simulink model "dcmotor_model"  (R2018b)
settings: Solver=ode15s  StartTime=0.0  StopTime=10.0  RelTol=1e-3  EnableMultiTasking=on
values from neighbouring files (symbols this model uses):
  fm = 7.2702e-06    [init.m]
  Imax = 10    [init.m]
  Jm = 2.7438e-06    [init.m]
  k = 43.8    [init.m]
  kM = 0.0054436    [init.m]
  L = 2.2223e-05    [init.m]
  R = 4.0191    [init.m]
settings Model: Creator=Akos  LastModifiedBy=akos
settings OptimizationCC: LifeSpan=inf
settings DebuggingCC: SFUnexpectedBacktrackingDiag=warning  SFNoUnconditionalDefaultTransitionDiag=warning
settings SFSimCC: SimUseLocalCustomCode=off
settings RTWCC: RTWUseLocalCustomCode=off
settings CodeAppCC: StateflowObjectComments=on
settings GRTTargetCC: TargetLangStandard=C89/C90 (ANSI)
settings ConfigComp: CovMetricSettings=dw  CovHtmlReporting=on  CovSaveCumulativeToWorkspaceVar=on  CovSaveSingleToWorkspaceVar=on  CovExternalEMLEnable=off

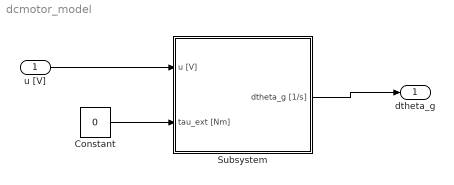
== system dcmotor_model ==
  u [V] : Inport
  Constant : Constant  Value=0
  Subsystem : Subsystem
  dtheta_g : Outport
  wires:
  u [V]/1 -> Subsystem/1(u [V])
  Constant/1 -> Subsystem/2(tau_ext [Nm])
  Subsystem/1(dtheta_g [1/s]) -> dtheta_g/1

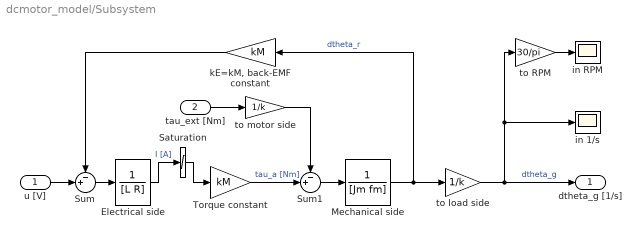
== system dcmotor_model/Subsystem ==
  u [V] : Inport
  tau_ext [Nm] : Inport  Port=2
  Electrical side : TransferFcn  Denominator=[L R]
  Mechanical side : TransferFcn  Denominator=[Jm fm]
  Saturation : Saturate  UpperLimit=Imax  LowerLimit=-Imax
  Sum : Sum  Inputs=-+|
  Sum1 : Sum  Inputs=-+|
  Torque constant : Gain  Gain=kM  SaturateOnIntegerOverflow=on  OutDataTypeStr=Inherit: Same as input  ParamDataTypeStr=Inherit: Same as input
  in 1/s : Scope
  in RPM : Scope
  "kE=kM, back-EMF constant" : Gain  Gain=kM  SaturateOnIntegerOverflow=on  OutDataTypeStr=Inherit: Same as input  ParamDataTypeStr=Inherit: Same as input
  to RPM : Gain  Gain=30/pi  SaturateOnIntegerOverflow=on  OutDataTypeStr=Inherit: Same as input  ParamDataTypeStr=Inherit: Same as input
  to load side : Gain  Gain=1/k  SaturateOnIntegerOverflow=on  OutDataTypeStr=Inherit: Same as input  ParamDataTypeStr=Inherit: Same as input
  to motor side : Gain  Gain=1/k  SaturateOnIntegerOverflow=on  OutDataTypeStr=Inherit: Same as input  ParamDataTypeStr=Inherit: Same as input
  dtheta_g [1/s] : Outport
  wires:
  tau_ext [Nm]/1 -> to motor side/1
  Sum/1 -> Electrical side/1
  to motor side/1 -> Sum1/1
  Torque constant/1 -> Sum1/2  "tau_a [Nm]"
  to load side/1 -> to RPM/1, in 1/s/1, dtheta_g [1/s]/1  "dtheta_g"
  "kE=kM, back-EMF constant"/1 -> Sum/1
  u [V]/1 -> Sum/2
  Sum1/1 -> Mechanical side/1
  Mechanical side/1 -> to load side/1, "kE=kM, back-EMF constant"/1  "dtheta_r"
  Electrical side/1 -> Saturation/1  "I [A]"
  to RPM/1 -> in RPM/1
  Saturation/1 -> Torque constant/1
